simulink model "MDS_interaction"  (R2020b)
settings: Solver=FixedStepAuto  StartTime=0  StopTime=10.0  FixedStep=0.001  MaxStep=0.05  RelTol=1e-3
values from neighbouring files (symbols this model uses):
  e_max = 0.01    [init.m]
  F_int_max = [5;5]    [init.m]
  F_max = [4;4]    [init.m]
  M = 1    [init.m]
  mass = 1    [init.m]
  ts_bound = 0.05    [init.m]
libraries: cstblocks x2
settings Model: Creator=chiara-s  LastModifiedBy=giorg

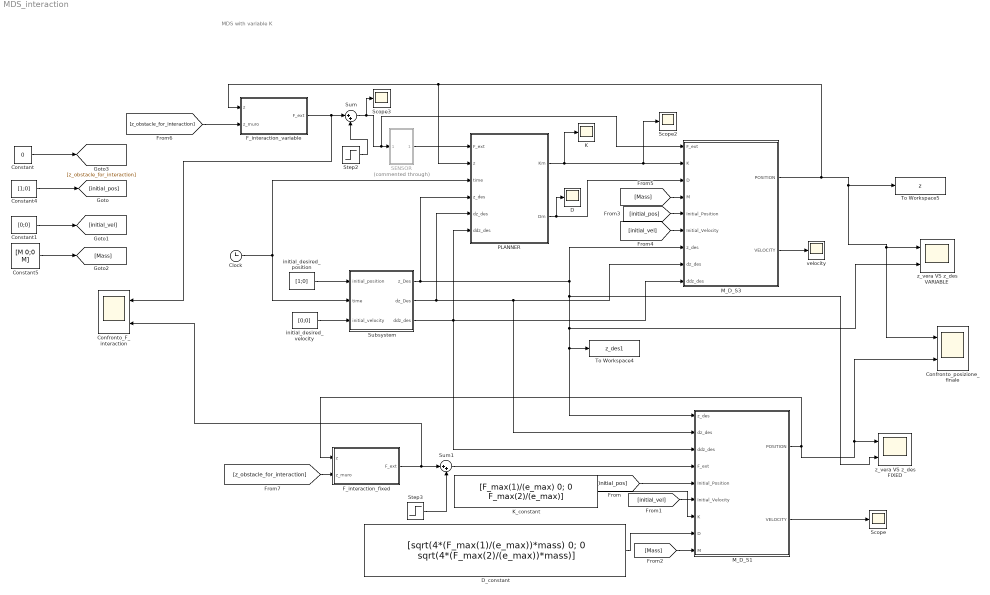
== system MDS_interaction ==
  note: MDS with variable K
  Clock : Clock
  Confronto_F_interaction : Scope  NumInputPorts=2
  Confronto_posizione_finale : Scope  NumInputPorts=2
  Constant : Constant  Value=0
  Constant1 : Constant  Value=[0;0]
  Constant4 : Constant  Value=[1;0]
  Constant5 : Constant  Value=[M 0;0 M]
  D : Scope
  D_constant : Constant  Value=[sqrt(4*(F_max(1)/(e_max))*mass) 0; 0 sqrt(4*(F_max(2)/(e_max))*mass)]
  F_interaction_fixed : MATLAB Function  TreatAsAtomicUnit=on
  F_interaction_variable : MATLAB Function  TreatAsAtomicUnit=on
  K : Scope
  K_constant : Constant  Value=[F_max(1)/(e_max) 0; 0 F_max(2)/(e_max)]
  M_D_S1 : Subsystem
  M_D_S3 : Subsystem
  PLANNER : MATLAB Function  TreatAsAtomicUnit=on
  SENSOR : Subsystem  Commented=through
  Scope : Scope
  Scope2 : Scope
  Scope3 : Scope
  Step2 : Step  Time=0  Before=[0;0]  After=[F_max(1);0]  SampleTime=0
  Step3 : Step  Time=0  Before=[0;0]  After=[F_max(1); 0]  SampleTime=0
  Subsystem : Subsystem
  Sum : Sum  Inputs=|++
  Sum1 : Sum  Inputs=|++
  To Workspace4 : ToWorkspace  VariableName=z_des1  SaveFormat=Structure With Time  SampleTime=-1
      settings: Save2DSignal=2-D array (concatenate along first dimension)
  To Workspace5 : ToWorkspace  VariableName=z  SaveFormat=Structure With Time  SampleTime=-1
  initial_desired_position : Constant  Value=[1;0]
  initial_desired_velocity : Constant  Value=[0;0]
  velocity : Scope
  z_vera VS z_des FIXED : Scope  NumInputPorts=2
  z_vera VS z_des VARIABLE : Scope  NumInputPorts=2
  wires:
  M_D_S3/1(POSITION) -> PLANNER/2(z), F_interaction_variable/1(z), Confronto_posizione_finale/1, z_vera VS z_des VARIABLE/1, To Workspace5/1
  Subsystem/1(z_Des) -> M_D_S3/7(z_des), M_D_S1/1(z_des), To Workspace4/1, z_vera VS z_des VARIABLE/2, z_vera VS z_des FIXED/2, PLANNER/4(z_des)
  PLANNER/2(Dm) -> M_D_S3/3(D), D/1
  F_interaction_variable/1(F_ext) -> Sum/1, Confronto_F_interaction/1
  SENSOR/1(Out1) -> PLANNER/1(F_ext)
  Clock/1 -> Subsystem/2(time), PLANNER/3(time)
  initial_desired_velocity/1 -> Subsystem/3(initial_velocity)
  initial_desired_position/1 -> Subsystem/1(initial_position)
  Subsystem/2(dz_Des) -> PLANNER/5(dz_des), M_D_S1/2(dz_des), M_D_S3/8(dz_des)
  Subsystem/3(ddz_des) -> M_D_S1/3(ddz_des), M_D_S3/9(ddz_des), PLANNER/6(ddz_des)
  M_D_S3/2(VELOCITY) -> velocity/1
  [z_obstacle_for_interaction] -> F_interaction_variable/2(z_muro)
  M_D_S1/1(POSITION) -> Confronto_posizione_finale/2, z_vera VS z_des FIXED/1, F_interaction_fixed/1(z)
  F_interaction_fixed/1(F_ext) -> Confronto_F_interaction/2, Sum1/1
  K_constant/1 -> M_D_S1/7(K)
  D_constant/1 -> M_D_S1/8(D)
  [initial_vel] -> M_D_S1/6(Initial_Velocity)
  [initial_pos] -> M_D_S1/5(Initial_Position)
  [Mass] -> M_D_S1/9(M)
  Constant1/1 -> [initial_vel]
  Constant4/1 -> [initial_pos]
  Constant5/1 -> [Mass]
  [initial_pos] -> M_D_S3/5(Initial_Position)
  [initial_vel] -> M_D_S3/6(Initial_Velocity)
  [Mass] -> M_D_S3/4(M)
  M_D_S1/2(VELOCITY) -> Scope/1
  Constant/1 -> [z_obstacle_for_interaction]
  [z_obstacle_for_interaction] -> F_interaction_fixed/2(z_muro)
  Sum/1 -> Scope3/1, M_D_S3/1(F_ext), SENSOR/1(In1)
  Step2/1 -> Sum/2
  Sum1/1 -> M_D_S1/4(F_ext)
  Step3/1 -> Sum1/2
  PLANNER/1(Km) -> Scope2/1, M_D_S3/2(K), K/1

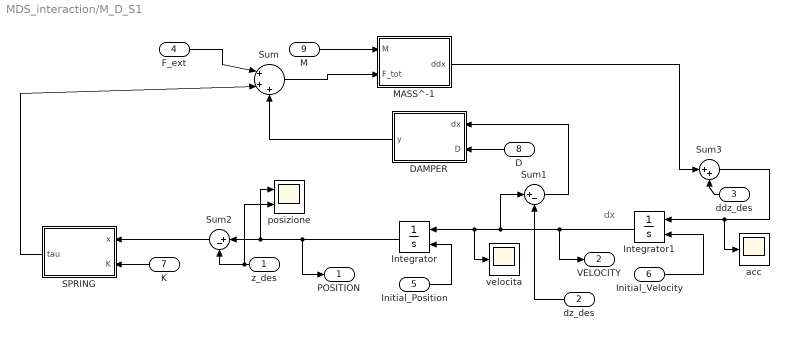
== system MDS_interaction/M_D_S1 ==
  note: dx
  z_des : Inport
  dz_des : Inport  Port=2
  ddz_des : Inport  Port=3
  F_ext : Inport  Port=4
  Initial_Position : Inport  Port=5
  Initial_Velocity : Inport  Port=6
  K : Inport  Port=7
  D : Inport  Port=8
  M : Inport  Port=9
  DAMPER : MATLAB Function  TreatAsAtomicUnit=on
  Integrator : Integrator  InitialConditionSource=external
  Integrator1 : Integrator  InitialConditionSource=external
  MASS^-1 : MATLAB Function  TreatAsAtomicUnit=on
  SPRING : MATLAB Function  TreatAsAtomicUnit=on
  Sum : Sum  Inputs=|+++
  Sum1 : Sum  Inputs=|+-
  Sum2 : Sum  Inputs=|+-
  Sum3 : Sum  Inputs=|++
  acc : Scope
  posizione : Scope  NumInputPorts=2
  velocita : Scope
  POSITION : Outport
  VELOCITY : Outport  Port=2
  wires:
  Integrator1/1 -> velocita/1, Integrator/1, Sum1/1, VELOCITY/1
  F_ext/1 -> Sum/1
  SPRING/1(tau) -> Sum/2
  Integrator/1 -> posizione/1, Sum2/1, POSITION/1
  DAMPER/1(y) -> Sum/3
  Sum/1 -> MASS^-1/2(F_tot)
  M/1 -> MASS^-1/1(M)
  D/1 -> DAMPER/2(D)
  K/1 -> SPRING/2(K)
  Initial_Velocity/1 -> Integrator1/2
  Initial_Position/1 -> Integrator/2
  z_des/1 -> posizione/2, Sum2/2
  Sum2/1 -> SPRING/1(x)
  dz_des/1 -> Sum1/2
  MASS^-1/1(ddx) -> Sum3/1
  Sum1/1 -> DAMPER/1(dx)
  ddz_des/1 -> Sum3/2
  Sum3/1 -> acc/1, Integrator1/1

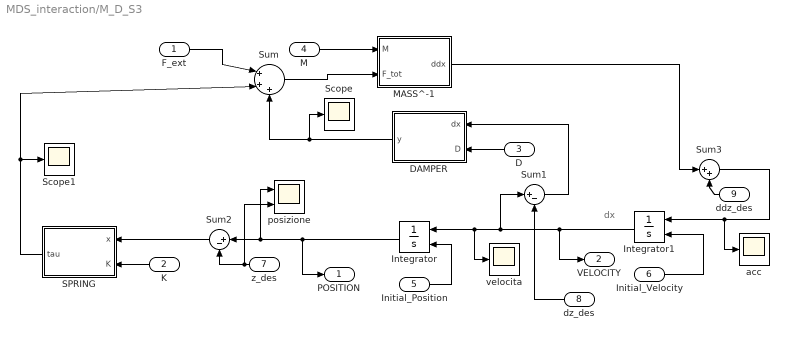
== system MDS_interaction/M_D_S3 ==
  note: dx
  F_ext : Inport
  K : Inport  Port=2
  D : Inport  Port=3
  M : Inport  Port=4
  Initial_Position : Inport  Port=5
  Initial_Velocity : Inport  Port=6
  z_des : Inport  Port=7
  dz_des : Inport  Port=8
  ddz_des : Inport  Port=9
  DAMPER : MATLAB Function  TreatAsAtomicUnit=on
  Integrator : Integrator  InitialConditionSource=external
  Integrator1 : Integrator  InitialConditionSource=external
  MASS^-1 : MATLAB Function  TreatAsAtomicUnit=on
  SPRING : MATLAB Function  TreatAsAtomicUnit=on
  Scope : Scope
  Scope1 : Scope
  Sum : Sum  Inputs=|+++
  Sum1 : Sum  Inputs=|+-
  Sum2 : Sum  Inputs=|+-
  Sum3 : Sum  Inputs=|++
  acc : Scope
  posizione : Scope  NumInputPorts=2
  velocita : Scope
  POSITION : Outport
  VELOCITY : Outport  Port=2
  wires:
  Integrator1/1 -> velocita/1, Integrator/1, Sum1/1, VELOCITY/1
  SPRING/1(tau) -> Sum/2, Scope1/1
  Integrator/1 -> posizione/1, Sum2/1, POSITION/1
  DAMPER/1(y) -> Scope/1, Sum/3
  Sum/1 -> MASS^-1/2(F_tot)
  M/1 -> MASS^-1/1(M)
  D/1 -> DAMPER/2(D)
  K/1 -> SPRING/2(K)
  Initial_Velocity/1 -> Integrator1/2
  Initial_Position/1 -> Integrator/2
  z_des/1 -> posizione/2, Sum2/2
  Sum2/1 -> SPRING/1(x)
  MASS^-1/1(ddx) -> Sum3/1
  Sum1/1 -> DAMPER/1(dx)
  Sum3/1 -> acc/1, Integrator1/1
  dz_des/1 -> Sum1/2
  ddz_des/1 -> Sum3/2
  F_ext/1 -> Sum/1

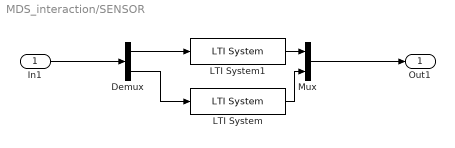
== system MDS_interaction/SENSOR ==
  In1 : Inport
  Demux : Demux  Outputs=2
  LTI System : cstblocks/LTI System  sys=tf(200^2,[1 0.5*2*200 200^2])  IC=[]
  LTI System1 : cstblocks/LTI System  sys=tf(200^2,[1 0.5*2*200 200^2])  IC=[]
  Mux : Mux  Inputs=2
  Out1 : Outport
  wires:
  LTI System1/1 -> Mux/1
  Demux/1 -> LTI System1/1
  Demux/2 -> LTI System/1
  LTI System/1 -> Mux/2
  Mux/1 -> Out1/1
  In1/1 -> Demux/1

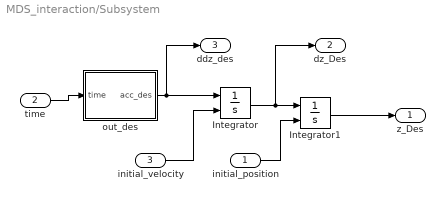
== system MDS_interaction/Subsystem ==
  initial_position : Inport
  time : Inport  Port=2
  initial_velocity : Inport  Port=3
  Integrator : Integrator  InitialConditionSource=external
  Integrator1 : Integrator  InitialConditionSource=external
  out_des : MATLAB Function  TreatAsAtomicUnit=on
  z_Des : Outport
  dz_Des : Outport  Port=2
  ddz_des : Outport  Port=3
  wires:
  Integrator1/1 -> z_Des/1
  time/1 -> out_des/1(time)
  Integrator/1 -> dz_Des/1, Integrator1/1
  out_des/1(acc_des) -> ddz_des/1, Integrator/1
  initial_velocity/1 -> Integrator/2
  initial_position/1 -> Integrator1/2

== matlab function MDS_interaction/Subsystem/out_des ==
  settings: sampleTime=0.1
  data: time input; acc_des output
function acc_des = fcn(time)
%% desired trajectory generator
if time < 0.1
    acc_des = [-5;0]; 
elseif time < 3.1
    acc_des = [0;0];
elseif time < 3.2
    acc_des = [5;0];
else 
    acc_des = [0;0];
end


end

== matlab function MDS_interaction/F_interaction_variable ==
  data: z input; F_ext output; z_muro input
function F_ext = fcn(z, z_muro)
% hypothesis: table reaction force with elastic behaviour
F_ext = zeros(2,1);
K = 10000;         % 1 mm displacement for 10 kg
F_ext(1) = 0;
F_ext(2) = 0;
% if contact is happened
if z_muro > z(1)
    F_ext(1) = K*(z_muro - z(1));
end

== matlab function MDS_interaction/M_D_S1/DAMPER ==
  data: dx input; y output; D input
function y = fcn(dx, D)
y = - D*dx;
end

== matlab function MDS_interaction/M_D_S1/MASS^-1 ==
  data: M input; ddx output; F_tot input
function ddx = fcn(M,F_tot)
ddx = (M^-1)*F_tot;
end

== matlab function MDS_interaction/M_D_S1/SPRING ==
  data: x input; tau output; K input
function tau = fcn(x, K)
tau= -K*x;
end

== matlab function MDS_interaction/F_interaction_fixed ==
  data: z input; F_ext output; z_muro input
function F_ext = fcn(z, z_muro)
% hypothesis: table reaction force with elastic behaviour
F_ext = zeros(2,1);
K = 10000;         % 1 mm displacement for 10 kg
F_ext(1) = 0;
F_ext(2) = 0;
% if contact is happened
if z_muro > z(1)
    F_ext(1) = K*(z_muro - z(1));
end

== matlab function MDS_interaction/M_D_S3/DAMPER ==
  data: dx input; y output; D input
function y = fcn(dx, D)
y = - D*dx;
end

== matlab function MDS_interaction/M_D_S3/MASS^-1 ==
  data: M input; ddx output; F_tot input
function ddx = fcn(M,F_tot)
ddx = (M^-1)*F_tot;
end

== matlab function MDS_interaction/M_D_S3/SPRING ==
  data: x input; tau output; K input
function tau = fcn(x, K)
tau= -K*x;
end

== matlab function MDS_interaction/PLANNER ==
  settings: updateMethod=DISCRETE
  data: F_max parameter; Km output; Dm output; e_max parameter; F_ext input; z input; time input; z_des input; dz_des input; ddz_des input; F_int_max parameter; mass parameter; ts_bound parameter
function [Km,Dm] = fcn(F_max, e_max,F_ext, z,time, z_des, dz_des, ddz_des, F_int_max, mass, ts_bound)

%% Description MDS_interaction
% decrease k after contact is sensed to limit the interaction force

%% Outputs
% Km            stiffness matrix
% Dm            damping matrix

%% Inputs
% time          current simulation time
% F_ext         measured external force
% mass          mass scalar value 
% F_int_max     desired interaction force
% z_des, dz_des, ddz_des                    desired trajectory
% z             current position
% F_max         estimated force disturbances
% e_max         maximum steady-state error

persistent F_prec kx ky dx dy t_changex t_changey t_settlx t_settly t_interaction

% time of a first interaction
if isempty(t_interaction)
    t_interaction = 1000;
end

% settling time
if isempty(t_settlx)
    t_settlx = 0;
end
if isempty(t_settly)
    t_settly = 0;
end

% time of last stiffness update
if isempty(t_changex)
    t_changex = 1000;
end
if isempty(t_changey)
    t_changey = 1000;
end

% previous measured force
if isempty(F_prec)
    F_prec = [0;0];
end

% initialization of k and d 
if isempty(kx)
   kx = F_max(1)/e_max; 
end
if isempty(ky)
   ky = F_max(2)/e_max;
end
if isempty(dx)
    dx = sqrt(4*kx*mass);
end
if isempty(dy)
    dy = sqrt(4*ky*mass);
end


if abs(F_ext(1)) > F_int_max(1) 
    % set t_interaction once contact is sensed
    if t_interaction == 1000
        t_interaction = time;
    end
    % if force is increasing
    if abs(F_prec(1)) < abs(F_ext(1))
        % if interaction force is higher than threshold
        if kx*abs(z(1)-z_des(1)) > F_int_max(1)
            % set k 
            kx = F_int_max(1)/abs(z(1)-z_des(1));
            % kx = 0.98*kx;
            dx = sqrt(4*kx*mass);

        end
    end
end
% Similarly for the other direction
if abs(F_ext(2)) > F_int_max(2) 
    if t_interaction == 1000
       t_interaction = time;
    end
    if abs(F_prec(2)) < abs(F_ext(2))
        if ky*abs(z(2)-z_des(2)) > F_int_max(2)
            ky = F_int_max(2)/abs(z(2)-z_des(2));
            % ky = 0.98*ky;
            dy = sqrt(4*ky*mass);
        end
    end
end

F_prec = F_ext;     % update for last force

% set final values 
Dm = diag([dx,dy]);
Km = diag([kx,ky]);
end
